simulink model "experiment_controller"  (R2023b)
settings: Solver=FixedStepAuto  StartTime=0.0  StopTime=27  FixedStep=par.Ta  RelTol=1e-3
InitFcn:
  | parameters
values from neighbouring files (symbols this model uses):
  param_robot = load_mu(param_robot, mu)    [parameters.m]
undefined symbols (not defined in the file or in its folder): filter_tau_p_slow_T_1, filter_tau_p_T_1, filter_tau_slow_T_1, filter_tau_T_1, filter_theta_p_slow_T_1, filter_theta_p_T_1, filter_theta_slow_T_1, par, param_controller, param_nullspace, sensor_torque_offset
libraries: simulink_extras x1
settings Model: TCT_ExtModeMexArgs=[169 254 109 124 1 1],16842784  SimulationMode=external  Creator=cha  LastModifiedBy=simon
settings SolverCC: AlgebraicLoopSolver=TrustRegion
settings OptimizationCC: LocalBlockOutputs=off
settings DebuggingCC: ReadBeforeWriteMsg=DisableAll  WriteAfterWriteMsg=DisableAll  WriteAfterReadMsg=DisableAll  MultiTaskDSMMsg=none  UnconnectedInputMsg=warning  UnconnectedOutputMsg=warning  UnconnectedLineMsg=warning  ArithmeticOperatorsInVariantConditions=warning
settings ModelReferenceCC: UpdateModelReferenceTargets=IfOutOfDate  EnableRefExpFcnMdlSchedulingChecks=on  EnableParallelModelReferenceBuilds=on
settings SFSimCC: SFSimEcho=off  SimUseLocalCustomCode=off  CustomCodeUndefinedFunction=UseInterfaceOnly  SimTargetLang=C++
settings RTWCC: Description=TwinCAT Target  SystemTargetFile=TwinCAT.tlc  GenCodeOnly=on  MakeCommand=make_tct  TemplateMakefile=tct_msbuild.tmf  GenerateReport=on  RTWUseLocalCustomCode=off  TargetLang=C++
settings RTWCC: CustomHeaderCode=|
  | #define fflush(stdout)
  | #define printf(...) m_spSrv->TcReportLog(ADSLOG_MSGTYPE_LOG,__VA_ARGS__)
settings CodeAppCC: MaxIdLength=47  StateflowObjectComments=on  MATLABSourceComments=on
settings STFCustomTargetCC: TargetLangStandard=C++03 (ISO)  CompOptLevelCompliant=on  MATLABClassNameForMDSCustomization=Simulink.SoftwareTarget.TargetSpecificTriggerConfigurationBase  GRTInterface=on  SystemTargetFile=TwinCAT.tlc

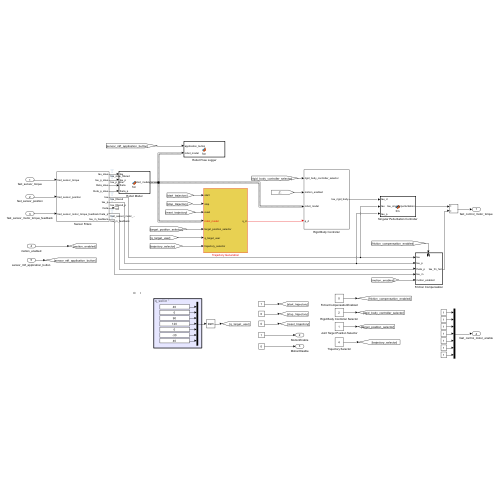
[thumbnail: Simulink's stored preview of the top-level diagram]
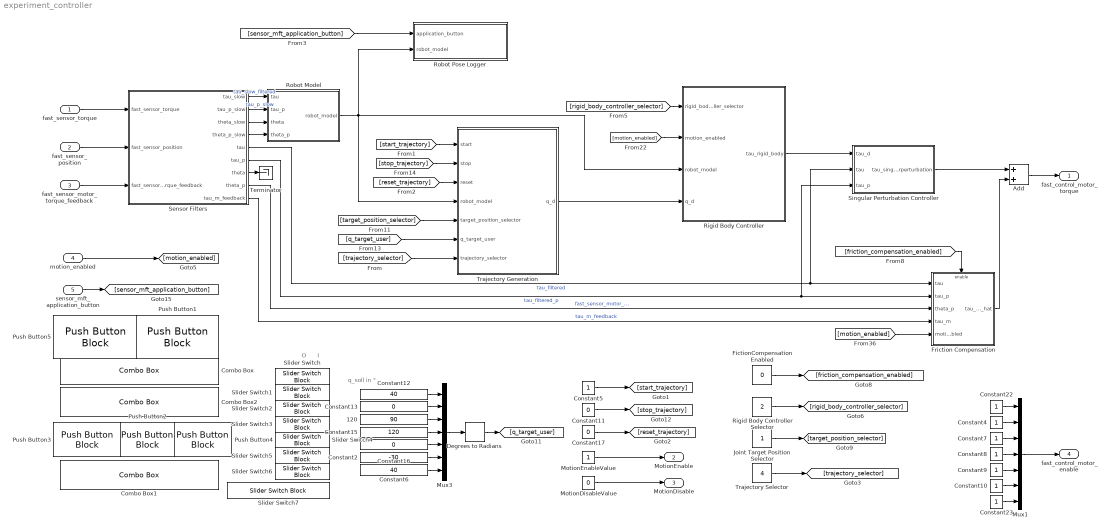
== system experiment_controller ==
  note: O
  note: q_soll in °
  note: I
  fast_sensor_torque : Inport
  fast_sensor_position : Inport  Port=2
  fast_sensor_motor_torque_feedback : Inport  Port=3
  motion_enabled : Inport  Port=4
  sensor_mft_application_button : Inport  Port=5
  120 : Constant  Value=90
  Add : Sum
  Combo Box : ComboBox  SelectedLabel=2: Joint-based I/O Linearization
      settings: Values={{'1: Gravity Compensation q-based', '2: Joint-based I/O Linearization'}, [1 2]}
  Combo Box1 : ComboBox  SelectedLabel=1: User defined position
      settings: Values={{'0: Candle position', '1: User defined position'}, [0 1]}
  Combo Box2 : ComboBox  SelectedLabel=4: Fourier Trajectory
      settings: Values={{'1: Start End Point', '2: Sinus Movement', '3: Spline Trajectory', '4: Fourier Trajectory'}, [1 2 3 4]}
  Constant{4..5,7..10,22..23} (8 alike) : Constant
  Constant{11,13,16..17} (4 alike) : Constant  Value=0
  Constant12 : Constant  Value=40
  Constant15 : Constant  Value=120
  Constant2 : Constant  Value=-30
  Constant6 : Constant  Value=40
  Degrees to Radians : simulink_extras/Transformations/Degrees to Radians
  FictionCompensationEnabled : Constant  Value=0
  Friction Compensation : Subsystem
  Joint Target Position Selector : Constant  OutDataTypeStr=uint32
  MotionDisableValue : Constant  Value=0
  MotionEnableValue : Constant
  Mux1 : Mux  Inputs=7
  Mux3 : Mux  Inputs=7
  Push Button1 : PushButtonBlock  ButtonText=Motion disable
  Push Button2 : PushButtonBlock  ButtonText=Stop trajectory  OffValue=0.000000
  Push Button3 : PushButtonBlock  ButtonText=Start trajectory  ButtonType=Latch  OffValue=0.000000
  Push Button4 : PushButtonBlock  ButtonText=Reset
  Push Button5 : PushButtonBlock  ButtonText=Motion enable  ButtonType=Latch  OffValue=0.000000
  Rigid Body Controller : Subsystem
  Rigid Body Controller Selector : Constant  Value=2  OutDataTypeStr=uint32
  Robot Model : MATLAB Function  TreatAsAtomicUnit=on
  Robot Pose Logger : MATLAB Function  TreatAsAtomicUnit=on
  Sensor Filters : Subsystem
  Singular Perturbation Controller : MATLAB Function  TreatAsAtomicUnit=on
  Slider Switch{,1..7} (8 alike) : SliderSwitchBlock  LabelPosition=Hide
  Terminator : Terminator
  Trajectory Generation : Subsystem
  Trajectory Selector : Constant  Value=4  OutDataTypeStr=uint32
  fast_control_motor_torque : Outport  VectorParamsAs1DForOutWhenUnconnected=off
  MotionEnable : Outport  Port=2  VectorParamsAs1DForOutWhenUnconnected=off
  MotionDisable : Outport  Port=3  VectorParamsAs1DForOutWhenUnconnected=off
  fast_control_motor_enable : Outport  Port=4  VectorParamsAs1DForOutWhenUnconnected=off
  wires:
  MotionEnableValue/1 -> MotionEnable/1
  MotionDisableValue/1 -> MotionDisable/1
  Sensor Filters/5(tau) -> Friction Compensation/1(tau), Singular Perturbation Controller/2(tau)  "tau_filtered"
  Mux1/1 -> fast_control_motor_enable/1
  Constant22/1 -> Mux1/1
  Constant4/1 -> Mux1/2
  Constant7/1 -> Mux1/3
  Constant8/1 -> Mux1/4
  Constant9/1 -> Mux1/5
  Constant10/1 -> Mux1/6
  Constant23/1 -> Mux1/7
  Singular Perturbation Controller/1(tau_singularperturbation) -> Add/1
  Sensor Filters/9(tau_m_feedback) -> Friction Compensation/4(tau_m)  "tau_m_feedback"
  Sensor Filters/6(tau_p) -> Friction Compensation/2(tau_p), Singular Perturbation Controller/3(tau_p)  "tau_filtered_p"
  Sensor Filters/8(theta_p) -> Friction Compensation/3(theta_p)  "fast_sensor_motor_..."
  Friction Compensation/1(tau_fm_hat) -> Add/2
  Constant5/1 -> [start_trajectory]
  Constant17/1 -> [reset_trajectory]
  [motion_enabled] -> Friction Compensation/5(motion_enabled)
  [motion_enabled] -> Rigid Body Controller/2(motion_enabled)
  [start_trajectory] -> Trajectory Generation/1(start)
  [reset_trajectory] -> Trajectory Generation/3(reset)
  [rigid_body_controller_selector] -> Rigid Body Controller/1(rigid_body_controller_selector)
  Rigid Body Controller Selector/1 -> [rigid_body_controller_selector]
  FictionCompensationEnabled/1 -> [friction_compensation_enabled]
  [friction_compensation_enabled] -> Friction Compensation/Enable
  Sensor Filters/7(theta) -> Terminator/1
  Joint Target Position Selector/1 -> [target_position_selector]
  [target_position_selector] -> Trajectory Generation/5(target_position_selector)
  Constant6/1 -> Mux3/7
  Constant12/1 -> Mux3/1
  Constant16/1 -> Mux3/5
  Mux3/1 -> Degrees to Radians/1
  Constant15/1 -> Mux3/4
  Constant13/1 -> Mux3/2
  Constant2/1 -> Mux3/6
  120/1 -> Mux3/3
  Constant11/1 -> [stop_trajectory]
  [stop_trajectory] -> Trajectory Generation/2(stop)
  Degrees to Radians/1 -> [q_target_user]
  Sensor Filters/1(tau_slow) -> Robot Model/1(tau)  "tau_slow_filtered"
  Sensor Filters/2(tau_p_slow) -> Robot Model/2(tau_p)  "tau_p_slow"
  Sensor Filters/3(theta_slow) -> Robot Model/3(theta)
  Sensor Filters/4(theta_p_slow) -> Robot Model/4(theta_p)
  [q_target_user] -> Trajectory Generation/6(q_target_user)
  [sensor_mft_application_button] -> Robot Pose Logger/1(application_button)
  Robot Model/1(robot_model) -> Rigid Body Controller/3(robot_model), Trajectory Generation/4(robot_model), Robot Pose Logger/2(robot_model)
  Trajectory Selector/1 -> [trajectory_selector]
  [trajectory_selector] -> Trajectory Generation/7(trajectory_selector)
  Rigid Body Controller/1(tau_rigid_body) -> Singular Perturbation Controller/1(tau_d)
  motion_enabled/1 -> [motion_enabled]
  sensor_mft_application_button/1 -> [sensor_mft_application_button]
  fast_sensor_motor_torque_feedback/1 -> Sensor Filters/3(fast_sensor_motor_torque_feedback)
  fast_sensor_position/1 -> Sensor Filters/2(fast_sensor_position)
  fast_sensor_torque/1 -> Sensor Filters/1(fast_sensor_torque)
  Add/1 -> fast_control_motor_torque/1
  Trajectory Generation/1(q_d) -> Rigid Body Controller/4(q_d)

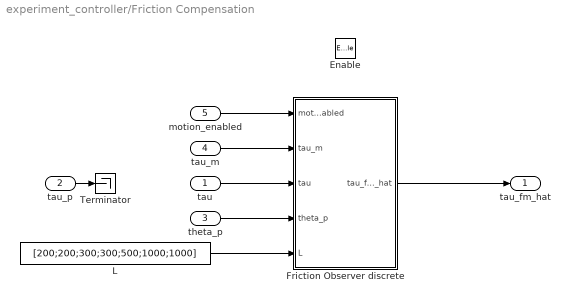
== system experiment_controller/Friction Compensation ==
  tau : Inport
  tau_p : Inport  Port=2
  theta_p : Inport  Port=3
  tau_m : Inport  Port=4
  motion_enabled : Inport  Port=5
  Enable : EnablePort
  Friction Observer discrete : MATLAB Function  TreatAsAtomicUnit=on
  L : Constant  Value=[200;200;300;300;500;1000;1000]
  Terminator : Terminator
  tau_fm_hat : Outport  VectorParamsAs1DForOutWhenUnconnected=off
  wires:
  L/1 -> Friction Observer discrete/5(L)
  tau_m/1 -> Friction Observer discrete/2(tau_m)
  Friction Observer discrete/1(tau_fm_hat) -> tau_fm_hat/1
  motion_enabled/1 -> Friction Observer discrete/1(motion_enabled)
  theta_p/1 -> Friction Observer discrete/4(theta_p)
  tau/1 -> Friction Observer discrete/3(tau)
  tau_p/1 -> Terminator/1

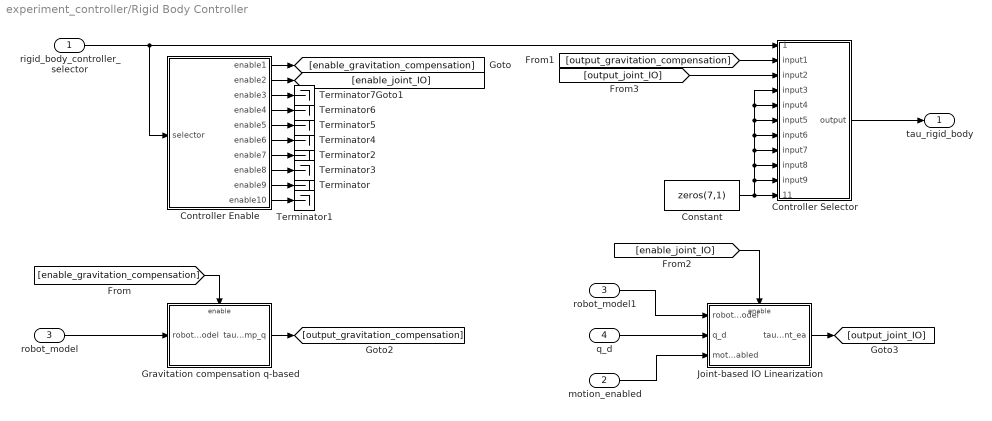
== system experiment_controller/Rigid Body Controller ==
  rigid_body_controller_selector : Inport
  motion_enabled : Inport  Port=2
  robot_model : Inport  Port=3
  q_d : Inport  Port=4
  Constant : Constant  Value=zeros(7,1)
  Controller Enable : MATLAB Function  TreatAsAtomicUnit=on
  Controller Selector : MATLAB Function  TreatAsAtomicUnit=on
  Gravitation compensation q-based : Subsystem
  Joint-based IO Linearization : Subsystem
  Terminator{,1..7} (8 alike) : Terminator
  robot_model1 : InportShadow  Port=3
  tau_rigid_body : Outport  VectorParamsAs1DForOutWhenUnconnected=off
  wires:
  Controller Selector/1(output) -> tau_rigid_body/1
  rigid_body_controller_selector/1 -> Controller Selector/1(selector), Controller Enable/1(selector)
  robot_model/1 -> Gravitation compensation q-based/1(robot_model)
  q_d/1 -> Joint-based IO Linearization/2(q_d)
  motion_enabled/1 -> Joint-based IO Linearization/3(motion_enabled)
  Controller Enable/9(enable9) -> Terminator/1
  Controller Enable/10(enable10) -> Terminator1/1
  Controller Enable/7(enable7) -> Terminator2/1
  Controller Enable/8(enable8) -> Terminator3/1
  Controller Enable/4(enable4) -> Terminator6/1
  Controller Enable/5(enable5) -> Terminator5/1
  Constant/1 -> Controller Selector/4(input3), Controller Selector/5(input4), Controller Selector/6(input5), Controller Selector/7(input6), Controller Selector/8(input7), Controller Selector/9(input8), Controller Selector/10(input9), Controller Selector/11(input10)
  Controller Enable/3(enable3) -> Terminator7/1
  robot_model1/1 -> Joint-based IO Linearization/1(robot_model)
  Controller Enable/1(enable1) -> [enable_gravitation_compensation]
  Controller Enable/2(enable2) -> [enable_joint_IO]
  [enable_gravitation_compensation] -> Gravitation compensation q-based/Enable
  Gravitation compensation q-based/1(tau_d_gravcomp_q) -> [output_gravitation_compensation]
  [output_gravitation_compensation] -> Controller Selector/2(input1)
  [enable_joint_IO] -> Joint-based IO Linearization/Enable
  Joint-based IO Linearization/1(tau_d_joint_ea) -> [output_joint_IO]
  [output_joint_IO] -> Controller Selector/3(input2)
  Controller Enable/6(enable6) -> Terminator4/1

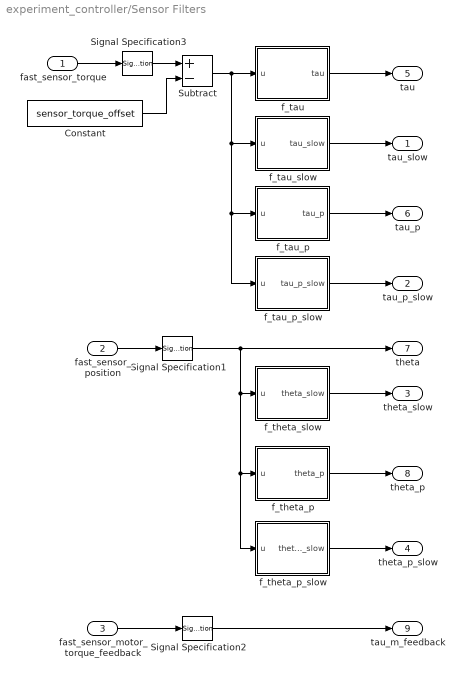
== system experiment_controller/Sensor Filters ==
  fast_sensor_torque : Inport
  fast_sensor_position : Inport  Port=2
  fast_sensor_motor_torque_feedback : Inport  Port=3
  Constant : Constant  Value=sensor_torque_offset
  Signal Specification1 : SignalSpecification  Dimensions=7
  Signal Specification2 : SignalSpecification  Dimensions=7
  Signal Specification3 : SignalSpecification  Dimensions=7
  Subtract : Sum  Inputs=+-
  f_tau : MATLAB Function  TreatAsAtomicUnit=on
  f_tau_p : MATLAB Function  TreatAsAtomicUnit=on
  f_tau_p_slow : MATLAB Function  TreatAsAtomicUnit=on
  f_tau_slow : MATLAB Function  TreatAsAtomicUnit=on
  f_theta_p : MATLAB Function  TreatAsAtomicUnit=on
  f_theta_p_slow : MATLAB Function  TreatAsAtomicUnit=on
  f_theta_slow : MATLAB Function  TreatAsAtomicUnit=on
  tau_slow : Outport  VectorParamsAs1DForOutWhenUnconnected=off
  tau_p_slow : Outport  Port=2  VectorParamsAs1DForOutWhenUnconnected=off
  theta_slow : Outport  Port=3  VectorParamsAs1DForOutWhenUnconnected=off
  theta_p_slow : Outport  Port=4  VectorParamsAs1DForOutWhenUnconnected=off
  tau : Outport  Port=5  VectorParamsAs1DForOutWhenUnconnected=off
  tau_p : Outport  Port=6  VectorParamsAs1DForOutWhenUnconnected=off
  theta : Outport  Port=7  VectorParamsAs1DForOutWhenUnconnected=off
  theta_p : Outport  Port=8  VectorParamsAs1DForOutWhenUnconnected=off
  tau_m_feedback : Outport  Port=9  VectorParamsAs1DForOutWhenUnconnected=off
  wires:
  fast_sensor_position/1 -> Signal Specification1/1
  fast_sensor_motor_torque_feedback/1 -> Signal Specification2/1
  f_theta_p/1(theta_p) -> theta_p/1
  Signal Specification1/1 -> theta/1, f_theta_slow/1(u), f_theta_p_slow/1(u), f_theta_p/1(u)
  f_tau_p/1(tau_p) -> tau_p/1
  f_theta_p_slow/1(theta_p_slow) -> theta_p_slow/1
  f_tau/1(tau) -> tau/1
  Signal Specification2/1 -> tau_m_feedback/1
  f_theta_slow/1(theta_slow) -> theta_slow/1
  f_tau_slow/1(tau_slow) -> tau_slow/1
  f_tau_p_slow/1(tau_p_slow) -> tau_p_slow/1
  Constant/1 -> Subtract/2
  Subtract/1 -> f_tau/1(u), f_tau_slow/1(u), f_tau_p_slow/1(u), f_tau_p/1(u)
  fast_sensor_torque/1 -> Signal Specification3/1
  Signal Specification3/1 -> Subtract/1

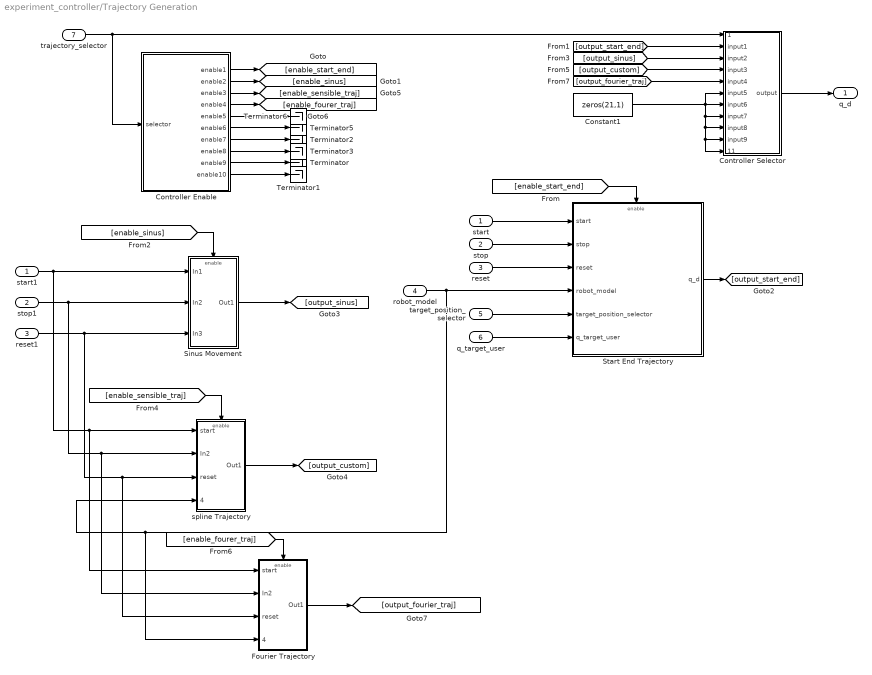
== system experiment_controller/Trajectory Generation ==
  start : Inport
  stop : Inport  Port=2
  reset : Inport  Port=3
  robot_model : Inport  Port=4
  target_position_selector : Inport  Port=5
  q_target_user : Inport  Port=6
  trajectory_selector : Inport  Port=7
  Constant1 : Constant  Value=zeros(21,1)
  Controller Enable : MATLAB Function  TreatAsAtomicUnit=on
  Controller Selector : MATLAB Function  TreatAsAtomicUnit=on
  Fourier Trajectory : Subsystem
  Sinus Movement : Subsystem
  Start End Trajectory : Subsystem
  Terminator{,1..3,5..6} (6 alike) : Terminator
  reset1 : InportShadow  Port=3
  spline Trajectory : Subsystem
  start1 : InportShadow
  stop1 : InportShadow  Port=2
  q_d : Outport  VectorParamsAs1DForOutWhenUnconnected=off
  wires:
  start/1 -> Start End Trajectory/1(start)
  reset/1 -> Start End Trajectory/3(reset)
  stop/1 -> Start End Trajectory/2(stop)
  robot_model/1 -> Fourier Trajectory/4(robot_model), spline Trajectory/4(robot_model), Start End Trajectory/4(robot_model)
  q_target_user/1 -> Start End Trajectory/6(q_target_user)
  target_position_selector/1 -> Start End Trajectory/5(target_position_selector)
  Controller Enable/4(enable4) -> [enable_fourer_traj]
  Constant1/1 -> Controller Selector/11(input10), Controller Selector/10(input9), Controller Selector/9(input8), Controller Selector/8(input7), Controller Selector/6(input5), Controller Selector/7(input6)
  Controller Enable/7(enable7) -> Terminator2/1
  Controller Enable/6(enable6) -> Terminator5/1
  Controller Enable/8(enable8) -> Terminator3/1
  Controller Enable/10(enable10) -> Terminator1/1
  [output_start_end] -> Controller Selector/2(input1)
  Controller Enable/9(enable9) -> Terminator/1
  Controller Enable/3(enable3) -> [enable_sensible_traj]
  Controller Enable/1(enable1) -> [enable_start_end]
  [enable_start_end] -> Start End Trajectory/Enable
  Controller Enable/2(enable2) -> [enable_sinus]
  Controller Selector/1(output) -> q_d/1
  Start End Trajectory/1(q_d) -> [output_start_end]
  trajectory_selector/1 -> Controller Enable/1(selector), Controller Selector/1(selector)
  [enable_sinus] -> Sinus Movement/Enable
  [output_sinus] -> Controller Selector/3(input2)
  Sinus Movement/1(Out1) -> [output_sinus]
  start1/1 -> Fourier Trajectory/1(start), spline Trajectory/1(start), Sinus Movement/1(In1)
  stop1/1 -> Fourier Trajectory/2(In2), spline Trajectory/2(In2), Sinus Movement/2(In2)
  reset1/1 -> Fourier Trajectory/3(reset), spline Trajectory/3(reset), Sinus Movement/3(In3)
  [enable_sensible_traj] -> spline Trajectory/Enable
  spline Trajectory/1(Out1) -> [output_custom]
  [output_custom] -> Controller Selector/4(input3)
  Controller Enable/5(enable5) -> Terminator6/1
  [enable_fourer_traj] -> Fourier Trajectory/Enable
  Fourier Trajectory/1(Out1) -> [output_fourier_traj]
  [output_fourier_traj] -> Controller Selector/5(input4)

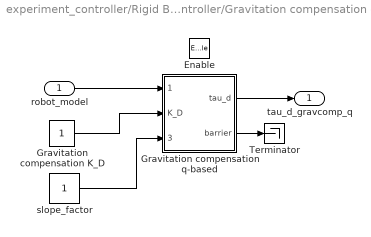
== system experiment_controller/Rigid Body Controller/Gravitation compensation q-based ==
  robot_model : Inport
  Enable : EnablePort  StatesWhenEnabling=reset
  Gravitation compensation q-based : MATLAB Function  TreatAsAtomicUnit=on
  Gravitation compensation K_D : Constant
  Terminator : Terminator
  slope_factor : Constant
  tau_d_gravcomp_q : Outport  VectorParamsAs1DForOutWhenUnconnected=off
  wires:
  robot_model/1 -> Gravitation compensation q-based/1(robot_model)
  Gravitation compensation q-based/1(tau_d) -> tau_d_gravcomp_q/1
  Gravitation compensation K_D/1 -> Gravitation compensation q-based/2(K_D)
  Gravitation compensation q-based/2(barrier) -> Terminator/1
  slope_factor/1 -> Gravitation compensation q-based/3(slope_factor)

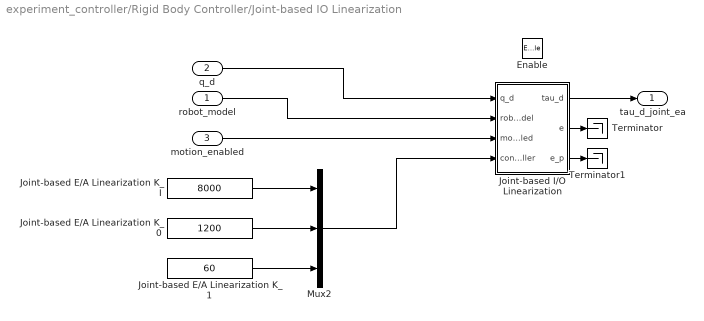
== system experiment_controller/Rigid Body Controller/Joint-based IO Linearization ==
  robot_model : Inport
  q_d : Inport  Port=2
  motion_enabled : Inport  Port=3
  Enable : EnablePort  StatesWhenEnabling=reset
  Joint-based E/A Linearization K_0 : Constant  Value=1200
  Joint-based E/A Linearization K_1 : Constant  Value=60
  Joint-based E/A Linearization K_I : Constant  Value=8000
  Joint-based I/O Linearization : MATLAB Function  TreatAsAtomicUnit=on
  Mux2 : Mux  Inputs=3
  Terminator : Terminator
  Terminator1 : Terminator
  tau_d_joint_ea : Outport  VectorParamsAs1DForOutWhenUnconnected=off
  wires:
  motion_enabled/1 -> Joint-based I/O Linearization/3(motion_enabled)
  Joint-based E/A Linearization K_I/1 -> Mux2/1
  Joint-based E/A Linearization K_1/1 -> Mux2/3
  Joint-based E/A Linearization K_0/1 -> Mux2/2
  Joint-based I/O Linearization/1(tau_d) -> tau_d_joint_ea/1
  q_d/1 -> Joint-based I/O Linearization/1(q_d)
  Mux2/1 -> Joint-based I/O Linearization/4(controller)
  robot_model/1 -> Joint-based I/O Linearization/2(robot_model)
  Joint-based I/O Linearization/2(e) -> Terminator/1
  Joint-based I/O Linearization/3(e_p) -> Terminator1/1

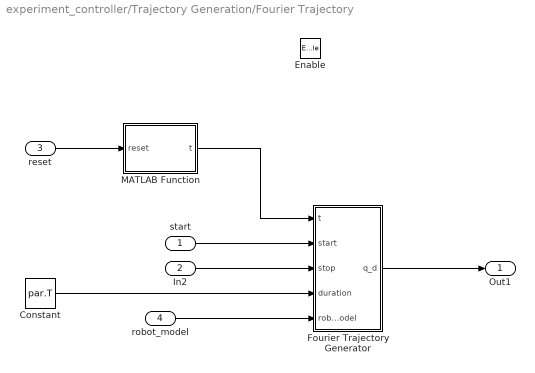
== system experiment_controller/Trajectory Generation/Fourier Trajectory ==
  start : Inport
  In2 : Inport  Port=2
  reset : Inport  Port=3
  robot_model : Inport  Port=4
  Enable : EnablePort  StatesWhenEnabling=reset
  Constant : Constant  Value=par.T
  Fourier Trajectory Generator : MATLAB Function  TreatAsAtomicUnit=on
  MATLAB Function : MATLAB Function  TreatAsAtomicUnit=on
  Out1 : Outport  VectorParamsAs1DForOutWhenUnconnected=off
  wires:
  Fourier Trajectory Generator/1(q_d) -> Out1/1
  start/1 -> Fourier Trajectory Generator/2(start)
  In2/1 -> Fourier Trajectory Generator/3(stop)
  reset/1 -> MATLAB Function/1(reset)
  Constant/1 -> Fourier Trajectory Generator/4(duration)
  MATLAB Function/1(t) -> Fourier Trajectory Generator/1(t)
  robot_model/1 -> Fourier Trajectory Generator/5(robot_model)

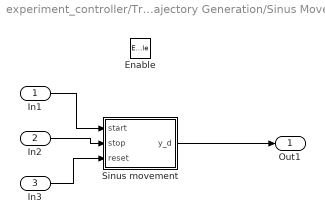
== system experiment_controller/Trajectory Generation/Sinus Movement ==
  In1 : Inport
  In2 : Inport  Port=2
  In3 : Inport  Port=3
  Enable : EnablePort  StatesWhenEnabling=reset
  Sinus movement : MATLAB Function  TreatAsAtomicUnit=on
  Out1 : Outport  VectorParamsAs1DForOutWhenUnconnected=off
  wires:
  Sinus movement/1(y_d) -> Out1/1
  In1/1 -> Sinus movement/1(start)
  In2/1 -> Sinus movement/2(stop)
  In3/1 -> Sinus movement/3(reset)

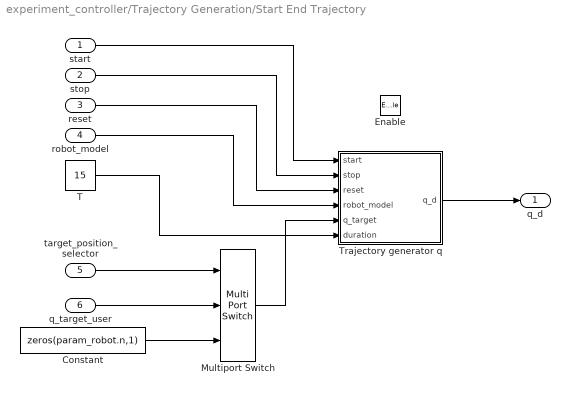
== system experiment_controller/Trajectory Generation/Start End Trajectory ==
  start : Inport
  stop : Inport  Port=2
  reset : Inport  Port=3
  robot_model : Inport  Port=4
  target_position_selector : Inport  Port=5
  q_target_user : Inport  Port=6
  Enable : EnablePort  StatesWhenEnabling=reset
  Constant : Constant  Value=zeros(param_robot.n,1)
  Multiport Switch : MultiPortSwitch  Inputs=2  DiagnosticForDefault=None  SaturateOnIntegerOverflow=off  InputSameDT=off
  T : Constant  Value=15
  Trajectory generator q : MATLAB Function  TreatAsAtomicUnit=on
  q_d : Outport  VectorParamsAs1DForOutWhenUnconnected=off
  wires:
  Trajectory generator q/1(q_d) -> q_d/1
  q_target_user/1 -> Multiport Switch/2
  Constant/1 -> Multiport Switch/3
  robot_model/1 -> Trajectory generator q/4(robot_model)
  target_position_selector/1 -> Multiport Switch/1
  T/1 -> Trajectory generator q/6(duration)
  stop/1 -> Trajectory generator q/2(stop)
  Multiport Switch/1 -> Trajectory generator q/5(q_target)
  reset/1 -> Trajectory generator q/3(reset)
  start/1 -> Trajectory generator q/1(start)

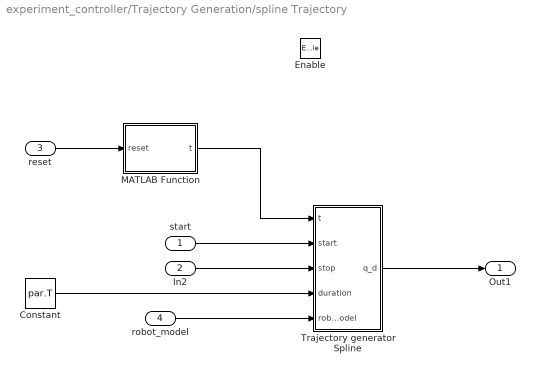
== system experiment_controller/Trajectory Generation/spline Trajectory ==
  start : Inport
  In2 : Inport  Port=2
  reset : Inport  Port=3
  robot_model : Inport  Port=4
  Enable : EnablePort  StatesWhenEnabling=reset
  Constant : Constant  Value=par.T
  MATLAB Function : MATLAB Function  TreatAsAtomicUnit=on
  Trajectory generator Spline : MATLAB Function  TreatAsAtomicUnit=on
  Out1 : Outport  VectorParamsAs1DForOutWhenUnconnected=off
  wires:
  Trajectory generator Spline/1(q_d) -> Out1/1
  start/1 -> Trajectory generator Spline/2(start)
  In2/1 -> Trajectory generator Spline/3(stop)
  reset/1 -> MATLAB Function/1(reset)
  Constant/1 -> Trajectory generator Spline/4(duration)
  MATLAB Function/1(t) -> Trajectory generator Spline/1(t)
  robot_model/1 -> Trajectory generator Spline/5(robot_model)

== matlab function experiment_controller/Trajectory Generation/Controller Selector ==
  data: selector input uint32; input1 input; input2 input; input3 input; input4 input; input5 input; input6 input; input7 input; input8 input; output output; input9 input; input10 input
function output = fcn(selector,input1,input2,input3,input4,input5,input6,input7,input8,input9,input10)
    switch selector
        case 1
            output=input1;
        case 2
            output=input2;
        case 3
            output=input3;
        case 4
            output=input4;
        case 5
            output=input5;
        case 6
            output=input6;
        case 7
            output=input7;
        case 8
            output=input8;
        case 9
            output=input9;
        case 10
            output=input10;
        otherwise
            output=zeros(size(input1));
    end
end

== matlab function experiment_controller/Trajectory Generation/Start End Trajectory/Trajectory generator q ==
  data: start input; stop input; reset input; robot_model input; q_d output; q_target input; duration input; param_controller parameter
function q_d = fcn(start,stop,reset,robot_model,q_target,duration,param_controller)
  persistent last_start;
  persistent last_stop;
  persistent started;
  persistent q__0;
  persistent q__T;
  persistent t;
  persistent T;
  
  if(isempty(last_start))
    last_start=0;
  end
  if(isempty(last_stop))
    last_stop=stop;
  end
  if(isempty(started))
    started=0;
  end
  if(isempty(t))
    t=0;
  end
  if(isempty(q__0))
    q__0=robot_model.q;
  end
  if(isempty(q__T))
    q__T=q_target;
  end
  if(isempty(T))
    T=duration;
  end
  
  if(reset)
    q__0=robot_model.q;
    q__T=q_target;
    T=duration;
    started=0;
    t=0;
  else
    if(started==1 && last_stop~=stop && stop==1)
      started=0;
    elseif(started==0 && last_start~=start && start==1)
      started=1;
    end
  end
  last_start=start;
  last_stop=stop;
  
  if(t<=0)
    q_d=[q__0;zeros(size(q__0));zeros(size(q__0))];
  elseif(t>=T)
    q_d=[q__T;zeros(size(q__T));zeros(size(q__T))];
  else
    t1 = (q__0 - q__T);
    t2 = 1 / T;
    t3 = (t ^ 2);
    t4 = (t2 ^ 2);
    t5 = (t2 * t4 ^ 2);
    t6 = (t * t2);
    t7 = (t - T);
    q_d = [q__0 + t * t3 * t2 * t4 * t1 * (t6 * (-6 * t6 + 15) - 10);...
      -30 * t3 * t1 * t7 ^ 2 * t5;...
      60 * t * t1 * t7 * (T - 2 * t) * t5];
  end
  if(started==1)
    t=t+param_controller.T_a;
  else
    %Hold last position, set velocity and acceleration zero
    n=7;
    q_d(n+1:end)=0;
  end
end

== matlab function experiment_controller/Robot Pose Logger ==
  data: application_button input; robot_model input
function fcn(application_button,robot_model)
  persistent last_application_button;

  if(isempty(last_application_button))
    last_application_button=application_button;
  end
  
  if(last_application_button~=application_button && application_button)
    fprintf('[%.10f,%.10f,%.10f,%.10f;%.10f,%.10f,%.10f,%.10f;%.10f,%.10f,%.10f,%.10f],...',...
      robot_model.H(1,1),robot_model.H(1,2),robot_model.H(1,3),robot_model.H(1,4),...
      robot_model.H(2,1),robot_model.H(2,2),robot_model.H(2,3),robot_model.H(2,4),...
      robot_model.H(3,1),robot_model.H(3,2),robot_model.H(3,3),robot_model.H(3,4));
  end
  
  last_application_button=application_button;
end

== matlab function experiment_controller/Trajectory Generation/spline Trajectory/MATLAB Function ==
  data: reset input; t output; par parameter
function t = fcn(reset, par)
    persistent ti;
  
  if(reset || isempty(ti))
    ti=0;
  end


  t = ti;
  ti=ti+par.Ta;
end

== matlab function experiment_controller/Sensor Filters/f_tau_slow ==
  data: u input; tau_slow output; param_controller parameter; filter_tau_slow_T_1 parameter
function tau_slow = func(u,param_controller, filter_tau_slow_T_1)
  persistent x;
  
  T_1=filter_tau_slow_T_1;
  alpha=exp(-param_controller.T_a./T_1);
  if(isempty(x))
    x=1./(1-alpha).*u;
    tau_slow=u;
  else
    tau_slow=(1-alpha).*x;
    x=alpha.*x+u;
  end
end

== matlab function experiment_controller/Trajectory Generation/Fourier Trajectory/MATLAB Function ==
  data: reset input; t output; par parameter
function t = fcn(reset, par)
    persistent ti;
  
  if(reset || isempty(ti))
    ti=0;
    t = 0;
  else 
      t = ti;
      ti=ti+par.Ta;
  end
end

== matlab function experiment_controller/Sensor Filters/f_theta_p ==
  data: u input; theta_p output; filter_theta_p_T_1 parameter; param_controller parameter
function theta_p = func(u,filter_theta_p_T_1,param_controller)
  persistent x;
  
  T_1=filter_theta_p_T_1;
  V=1/param_controller.T_a*(1-exp(-param_controller.T_a./T_1));
  if(isempty(x))
    x=-V.*u;
    theta_p=zeros(size(u));
  else
    theta_p=x+V.*u;
    x=exp(-param_controller.T_a./T_1).*x+(exp(-param_controller.T_a./T_1)-1).*V.*u;
  end
end

== matlab function experiment_controller/Trajectory Generation/Fourier Trajectory/Fourier Trajectory Generator ==
  data: t input; start input; stop input; duration input; q_d output; robot_model input; par parameter
function q_d = fcn(t,start,stop,duration, robot_model, par)
  persistent last_start;
  persistent last_stop;
  persistent started;
  persistent t_0;
  persistent q__0;
  persistent T;
  persistent a_params;
  persistent b_params;
  %persistent w;

  %if (isempty(w))
  w = 2* pi/duration;
  %end

  if (isempty(a_params)) 
    a_params = par.a;
  end

  if (isempty(b_params))
     b_params = par.b;
  end
  
  if(isempty(last_start))
    last_start=0;
  end
  if(isempty(last_stop))
    last_stop=stop;
  end
  if(isempty(started))
    started=0;
  end
  if(isempty(t_0))
    t_0=0;
  end
  if(isempty(q__0))
    q__0=robot_model.q;
  end
  if(isempty(T))
    T=duration;
  end
  
  if(started==1 && last_stop~=stop && stop==1)
    started=0;
    %Hold last position
  elseif(started==0 && last_start~=start && start==1)
    started=1;
    t_0=t;
    T=duration;
  end
  la.st_start=start;
  last_stop=stop;
  
  theta=(t-t_0)/T;
  theta_p=1/T;
  theta_pp=0;
  theta_limit=max(min(theta,1-1e-6),0);

  if(theta==theta_limit && started)
    q = zeros(7,1);
    qp = zeros(7,1);
    qpp = zeros(7,1);

    a_size = size(a_params);

    for i = 1:a_size(1)
        for l = 1:a_size(2)
            q(i) = q(i) + a_params(i,l) * sin(w * l * t) / (w*l) - b_params(i,l)*cos(w*l*t)/(w*l);
            qp(i) = qp(i) + a_params(i,l) * cos(w * l * t) + b_params(i,l)*sin(w*l*t);
            qpp(i) = qpp(i) - a_params(i,l) * sin(w * l * t) * (w*l) + b_params(i,l)*cos(w*l*t) * (w*l);
        end
    end
  else
    started=0;
    q=q__0;
    qp=zeros(size(q__0));
    qpp=zeros(size(q__0));
  end
  
  q_d=[q; qp; qpp];
  %q_d=zeros(21, 1);
end

== matlab function experiment_controller/Robot Model ==
  data: tau input; tau_p input; theta input; robot_model output Bus: robot_model; theta_p input; param_robot parameter; param_controller parameter
function robot_model = fcn(tau,tau_p,theta,theta_p,param_robot,param_controller)
  K=param_robot.K;
  
  robot_model=struct();
  %The calculation of q and q_p has to be performed with consistent cutoff
  %frequencies for the corresponding filters. The filters for q, q_p, tau
  %and tau_p have to have the same cutoff frequency.
  q=theta-diag(K).\tau;
  q_p=theta_p-diag(K).\tau_p;
  robot_model.q=q;                  % generalized coordinates
  robot_model.q_p=q_p;              % time derivative of generalized coordinates
  robot_model.theta=theta;          % motor angles
  robot_model.theta_p=theta_p;      % time derivative of motor angles
  %Path Following Control with reverse kinematic
  robot_model.H=hom_transform_endeffector(q,param_robot);               % homogenous transformation to end-effector
  robot_model.J=geo_jacobian_endeffector(q,param_robot);                % geometric jacobian to end-effector
  robot_model.J_p=geo_jacobian_endeffector_p(q,q_p,param_robot);        % time derivative of geometric jacobian to end-effector
  %If the singular perturbation controller is selected, the mass matrix has
  %to be modified according to Ott2008, Eq. (5.28).
  robot_model.M=inertia_matrix(q,param_robot);                          % rigid body inertia matrix
  %More efficient implementation for M+(I+K_tau)\B with diagonal
  %matrices K_tau and B: Only handle the diagonal elements.
  robot_model.M=robot_model.M+diag((1+param_controller.singular_perturbation.K_tau).\diag(param_robot.B));
  robot_model.C=coriolis_matrix(q,q_p,param_robot);                     % coriolis matrix
  robot_model.g=gravitational_forces(q,param_robot);                    % gravitational forces
end

== matlab function experiment_controller/Friction Compensation/Friction Observer discrete ==
  settings: sampleTime=param.T_a
  data: motion_enabled input; tau_m input; tau input; theta_p input; tau_fm_hat output; param_robot parameter; L input; param_controller parameter
function tau_fm_hat   = fcn(motion_enabled,tau_m,tau,theta_p, param_robot,L, param_controller)
  persistent x_theta_p_hat;

  if(isempty(x_theta_p_hat))
    x_theta_p_hat=zeros(param_robot.n,1);
  end
  
  if(motion_enabled)
    %Estimated, unmodeled friction
    tau_fm_hat=-L.*diag(param_robot.B).*(theta_p-x_theta_p_hat);
    %The term tau_m is the feedback torque from the motor. It contains the
    %added "tau_fm_hat", therefore it has to be subtracted, before feeding
    %it into the observer.
    %Notice, that not the actual control value is used, but the sensor
    %value from the motor. The latter signal is very, very noisy (standard
    %deviation of about 3 Nm at rest), but it shows the best behaviour for
    %estimating friction. It is also convenient, that the sensor value
    %implicitly contains the low-level saturation of the commanded value.
    x_theta_p_hat=x_theta_p_hat+param_controller.T_a*(diag(param_robot.B).\(tau_m-tau-tau_fm_hat));
  else
    x_theta_p_hat=zeros(param_robot.n,1);
    tau_fm_hat=zeros(param_robot.n,1);
  end
end

== matlab function experiment_controller/Sensor Filters/f_theta_slow ==
  data: u input; theta_slow output; param_controller parameter; filter_theta_slow_T_1 parameter
function theta_slow = func(u,param_controller, filter_theta_slow_T_1)
  persistent x;
  
  T_1=filter_theta_slow_T_1;
  alpha=exp(-param_controller.T_a./T_1);
  if(isempty(x))
    x=1./(1-alpha).*u;
    theta_slow=u;
  else
    theta_slow=(1-alpha).*x;
    x=alpha.*x+u;
  end
end

== matlab function experiment_controller/Sensor Filters/f_tau_p_slow ==
  data: u input; tau_p_slow output; filter_tau_p_slow_T_1 parameter; param_controller parameter
function tau_p_slow = func(u,filter_tau_p_slow_T_1,param_controller)
  persistent x;
  
  T_1=filter_tau_p_slow_T_1;
  V=1/param_controller.T_a*(1-exp(-param_controller.T_a./T_1));
  if(isempty(x))
    x=-V.*u;
    tau_p_slow=zeros(size(u));
  else
    tau_p_slow=x+V.*u;
    x=exp(-param_controller.T_a./T_1).*x+(exp(-param_controller.T_a./T_1)-1).*V.*u;
  end
end

== matlab function experiment_controller/Sensor Filters/f_theta_p_slow ==
  data: u input; theta_p_slow output; filter_theta_p_slow_T_1 parameter; param_controller parameter
function theta_p_slow = func(u,filter_theta_p_slow_T_1,param_controller)
  persistent x;
  
  T_1=filter_theta_p_slow_T_1;
  V=1/param_controller.T_a*(1-exp(-param_controller.T_a./T_1));
  if(isempty(x))
    x=-V.*u;
    theta_p_slow=zeros(size(u));
  else
    theta_p_slow=x+V.*u;
    x=exp(-param_controller.T_a./T_1).*x+(exp(-param_controller.T_a./T_1)-1).*V.*u;
  end
end

== matlab function experiment_controller/Rigid Body Controller/Controller Enable ==
  data: enable1 output; enable2 output; enable3 output; enable4 output; enable5 output; enable6 output; enable7 output; enable8 output; selector input uint32; enable9 output; enable10 output
function [enable1,enable2,enable3,enable4,enable5,enable6,enable7,enable8,enable9,enable10] = fcn(selector)
    enable1=(selector==1);
    enable2=(selector==2);
    enable3=(selector==3);
    enable4=(selector==4);
    enable5=(selector==5);
    enable6=(selector==6);
    enable7=(selector==7);
    enable8=(selector==8);
    enable9=(selector==9);
    enable10=(selector==10);
end

== matlab function experiment_controller/Rigid Body Controller/Controller Selector ==
  data: selector input uint32; input1 input; input2 input; input3 input; input4 input; input5 input; input6 input; input7 input; input8 input; output output; input9 input; input10 input
function output = fcn(selector,input1,input2,input3,input4,input5,input6,input7,input8,input9,input10)
    switch selector
        case 1
            output=input1;
        case 2
            output=input2;
        case 3
            output=input3;
        case 4
            output=input4;
        case 5
            output=input5;
        case 6
            output=input6;
        case 7
            output=input7;
        case 8
            output=input8;
        case 9
            output=input9;
        case 10
            output=input10;
        otherwise
            output=zeros(size(input1));
    end
end

== matlab function experiment_controller/Trajectory Generation/spline Trajectory/Trajectory generator Spline ==
  data: t input; start input; stop input; duration input; q_d output; param_trajectory_generator_spline parameter; robot_model input
function q_d = fcn(t,start,stop,duration,param_trajectory_generator_spline, robot_model)
  persistent last_start;
  persistent last_stop;
  persistent started;
  persistent t_0;
  persistent q__0;
  persistent T;
  
  if(isempty(last_start))
    last_start=0;
  end
  if(isempty(last_stop))
    last_stop=stop;
  end
  if(isempty(started))
    started=0;
  end
  if(isempty(t_0))
    t_0=0;
  end
  if(isempty(q__0))
    q__0=robot_model.q;
  end
  if(isempty(T))
    T=duration;
  end
  
  if(started==1 && last_stop~=stop && stop==1)
    started=0;
    %Hold last position
  elseif(started==0 && last_start~=start && start==1)
    started=1;
    t_0=t;
    T=duration;
  end
  la.st_start=start;
  last_stop=stop;
  
  theta=(t-t_0)/T;
  theta_p=1/T;
  theta_pp=0;
  theta_limit=max(min(theta,1-1e-6),0);

  if(theta==theta_limit && started)
    degree=3;
    %B-Spline basis functions
    i=bspline_findspan(theta_limit,param_trajectory_generator_spline);
    N=bspline_basisfunction(theta_limit,i,2,param_trajectory_generator_spline);
    q=sum(param_trajectory_generator_spline.position(i:i+degree,:).*repmat(N(1,1:degree+1)',[1,7]),1)';
    dq=sum(param_trajectory_generator_spline.position(i:i+degree,:).*repmat(N(2,1:degree+1)',[1,7]),1)';
    ddq=sum(param_trajectory_generator_spline.position(i:i+degree,:).*repmat(N(3,1:degree+1)',[1,7]),1)';
    
    q__0=q;
  else
    started=0;
    q=q__0;
    dq=zeros(size(q__0));
    ddq=zeros(size(q__0));
  end
  
  q_d=[q;
    dq*theta_p;
    ddq*theta_p^2+dq*theta_pp];
end

== matlab function experiment_controller/Rigid Body Controller/Gravitation compensation q-based/Gravitation compensation q-based ==
  data: robot_model input; tau_d output; K_D input; slope_factor input; param_nullspace parameter; barrier output; param_robot parameter
function [tau_d,barrier] = fcn(robot_model, K_D,slope_factor,param_nullspace,param_robot)
  n=param_robot.n;
  %% Barrier or penalty functions for nullspace controller
  %Desired position for nullspace
  p_1=...
    slope_factor*param_nullspace.q_limit_slope(1:n)./...
      (1./(param_nullspace.q_limit_range(1:n).^2)...
      -1./((param_nullspace.q_limit_upper(1:n)-param_nullspace.q_limit_lower(1:n)-param_nullspace.q_limit_range(1:n)).^2));
    
  q=robot_model.q;
  barrier=zeros(size(q));
  valid=q<param_nullspace.q_limit_upper(1:n) & q>param_nullspace.q_limit_lower(1:n);
  inside=q<(param_nullspace.q_limit_upper(1:n)-param_nullspace.q_limit_range(1:n)) & ...
    q>(param_nullspace.q_limit_lower(1:n)+param_nullspace.q_limit_range(1:n));
  barrier(valid)=(1./(q(valid)-param_nullspace.q_limit_upper(valid)).^2 ...
      -1./(param_nullspace.q_limit_lower(valid)-q(valid)).^2).*p_1(valid)...
    -slope_factor*param_nullspace.q_limit_slope(valid).*sign(q(valid));
  barrier(~valid)=NaN;
  barrier(inside)=0;
  
  tau_d=robot_model.g-K_D*robot_model.q_p-barrier;
end

== matlab function experiment_controller/Trajectory Generation/Sinus Movement/Sinus movement ==
  data: y_d output; start input; stop input; reset input; par parameter
function y_d = fcn(start,stop,reset,par)

persistent last_start;
persistent last_stop;
persistent started;
persistent t;

if(isempty(last_start))
    last_start=start;
end
if(isempty(last_stop))
    last_stop=stop;
end
if(isempty(started))
    started=0;
end
if(isempty(t))
    t=0;
end

if(reset)
    started=0;
    t=0;
else
    if(started==1 && last_stop~=stop && stop==1)
        started=0;
    elseif(started==0 && last_start~=start && start==1)
        started=1;
    end
end
last_start=start;
last_stop=stop;

if(started==1)
    t=t+par.Ta;
else
    t=0;
end

q = sin(2*pi/10*t);
q_p = sin(2*pi/10*t);
q_pp = sin(2*pi/10*t);

y_d=[repmat(q,7,1);repmat(q_p,7,1);repmat(q_pp,7,1)];

end

== matlab function experiment_controller/Sensor Filters/f_tau ==
  data: u input; tau output; param_controller parameter; filter_tau_T_1 parameter
function tau = func(u,param_controller, filter_tau_T_1)
  persistent x;
  
  T_1=filter_tau_T_1;
  alpha=exp(-param_controller.T_a./T_1);
  if(isempty(x))
    x=1./(1-alpha).*u;
    tau=u;
  else
    tau=(1-alpha).*x;
    x=alpha.*x+u;
  end
end

== matlab function experiment_controller/Sensor Filters/f_tau_p ==
  data: u input; tau_p output; filter_tau_p_T_1 parameter; param_controller parameter
function tau_p = func(u,filter_tau_p_T_1,param_controller)
  persistent x;
  
  T_1=filter_tau_p_T_1;
  V=1/param_controller.T_a*(1-exp(-param_controller.T_a./T_1));
  if(isempty(x))
    x=-V.*u;
    tau_p=zeros(size(u));
  else
    tau_p=x+V.*u;
    x=exp(-param_controller.T_a./T_1).*x+(exp(-param_controller.T_a./T_1)-1).*V.*u;
  end
end

== matlab function experiment_controller/Rigid Body Controller/Joint-based IO Linearization/Joint-based I//O Linearization ==
  data: q_d input; robot_model input; motion_enabled input; tau_d output; param_robot parameter; controller input; param_controller parameter; e output; e_p output
function [tau_d,e,e_p] = fcn(q_d,robot_model,motion_enabled, param_robot,controller,param_controller)
  persistent e_I;
  
  if(~motion_enabled || isempty(e_I))
    e_I=zeros(param_robot.n,1);
  end
  
  q_pp_d=q_d(2*param_robot.n+1:3*param_robot.n);
  q_p_d=q_d(param_robot.n+1:2*param_robot.n);
  q_d=q_d(1:param_robot.n);
  
  K_I=controller(1)*ones(param_robot.n,1);
  K_0=controller(2)*ones(param_robot.n,1);
  K_1=controller(3)*ones(param_robot.n,1);
  
  q=robot_model.q;
  q_p=robot_model.q_p;
  
  %Common "Computed Torque" equations
  M=robot_model.M;
  C=robot_model.C;
  g=robot_model.g;
  n=C*q_p+g;

  e=q-q_d;
  e_p=q_p-q_p_d;
  v=q_pp_d-K_1.*e_p-K_0.*e-K_I.*e_I;
  
  tau_d=M*v+n;
  
  e_I=e_I+e*param_controller.T_a;
end

== matlab function experiment_controller/Singular Perturbation Controller ==
  data: tau_d input; tau input; tau_p input; tau_singularperturbation output; param_controller parameter
function tau_singularperturbation  = fcn(tau_d,tau,tau_p,param_controller)
  %Implementation is taken from Ott 2008, chapter 5.4.
  tau_singularperturbation_controller_K=-param_controller.singular_perturbation.K_tau.*(tau-tau_d);
  tau_singularperturbation_controller_D=-param_controller.singular_perturbation.D_tau.*tau_p;
  tau_singularperturbation_controller=tau_singularperturbation_controller_K...
    +tau_singularperturbation_controller_D;
  tau_singularperturbation=tau_d+tau_singularperturbation_controller;
end

== matlab function experiment_controller/Trajectory Generation/Controller Enable ==
  data: enable1 output; enable2 output; enable3 output; enable4 output; enable5 output; enable6 output; enable7 output; enable8 output; selector input uint32; enable9 output; enable10 output
function [enable1,enable2,enable3,enable4,enable5,enable6,enable7,enable8,enable9,enable10] = fcn(selector)
    enable1=(selector==1);
    enable2=(selector==2);
    enable3=(selector==3);
    enable4=(selector==4);
    enable5=(selector==5);
    enable6=(selector==6);
    enable7=(selector==7);
    enable8=(selector==8);
    enable9=(selector==9);
    enable10=(selector==10);
end
